simulink model "zynq_7000_tutorial_3"  (R2023b)
settings: Solver=FixedStepDiscrete  StartTime=0.0  StopTime=10.0  RelTol=1e-3
PostLoadFcn:
  | zynq7000.setModelProperties(bdroot)
undefined symbols (not defined in the file): AXI_VDMA, B, cam_init, G, init_cam, out1, out2, out3, OV5640, PS_GPIO, PS_IIC, R, read_cam_rgb, ScuGicInterruptController, VideoOutput
libraries: waijung2_utilities_lib x2, deeplib x1, zynq7000_device_config_lib x1
Description:
  | This model is created using Waijung 2
  | (Version: 23.5a)
settings Model: Creator=Aimagin  LastModifiedBy=Chris
settings SolverCC: PositivePriorityOrder=on  AutoInsertRateTranBlk=on
settings OptimizationCC: DefaultParameterBehavior=Inlined  EnhancedBackFolding=on  PassReuseOutputArgsAs=Individual arguments  ZeroExternalMemoryAtStartup=off  ZeroInternalMemoryAtStartup=off  OptimizeBlockOrder=speed  DifferentSizesBufferReuse=on  OptimizationCustomize=off  EfficientTunableParamExpr=on
settings DebuggingCC: ParameterTunabilityLossMsg=error
settings HardwareCC: ProdBitPerPointer=32  ProdBitPerSizeT=32  ProdBitPerPtrDiffT=32  ProdLargestAtomicInteger=Long  ProdLargestAtomicFloat=Double  ProdWordSize=32  ProdHWDeviceType=ARM Compatible->ARM Cortex
settings ModelReferenceCC: EnableRefExpFcnMdlSchedulingChecks=on
settings SFSimCC: MATLABDynamicMemAlloc=off
settings RTWCC: Description=Waijung 2 ZYNQ7000 target  SystemTargetFile=zynq7000.tlc  TemplateMakefile=zynq7000.tmf  RetainRTWFile=on  TargetLang=C++  DLTargetLibrary=arm-compute  DLArmComputeArch=armv7
settings CodeAppCC: ForceParamTrailComments=on  IgnoreCustomStorageClasses=off  OperatorAnnotations=on  SimulinkDataObjDesc=on  SFDataObjDesc=on  InsertBlockDesc=on
settings STFCustomTargetCC: TargetLangStandard=C++11 (ISO)  MultiwordLength=256  GenerateSampleERTMain=on  ModelReferenceCompliant=off  CombineOutputUpdateFcns=on  ERTCustomFileBanners=on  SupportContinuousTime=off  SupportNonInlinedSFcns=off  RemoveResetFunc=on  SupportVariableSizeSignals=on  MATLABClassNameForMDSCustomization=Simulink.SoftwareTarget.ERTCustomization  SystemTargetFile=zynq7000.tlc
settings ERTTargetCC: TargetLangStandard=C++11 (ISO)  GenerateSampleERTMain=on  ModelReferenceCompliant=off  ParMdlRefBuildCompliant=off  CompOptLevelCompliant=off  ConcurrentExecutionCompliant=off  SupportVariableSizeSignals=on  ModelStepFunctionPrototypeControlCompliant=off  CPPClassGenCompliant=off  UseToolchainInfoCompliant=off  InlinedParameterPlacement=NonHierarchical  ERTSrcFileBannerTemplate=zynq7000_code_template.cgt  ERTHdrFileBannerTemplate=zynq7000_code_template.cgt  ERTDataSrcFileTemplate=zynq7000_code_template.cgt  ERTDataHdrFileTemplate=zynq7000_code_template.cgt  ERTCustomFileTemplate=zynq7000_file_process.tlc

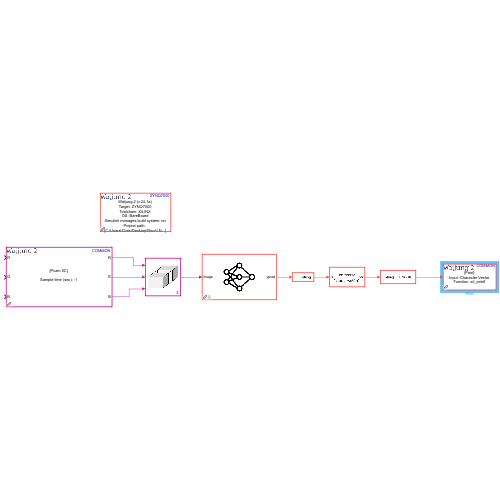
[thumbnail: Simulink's stored preview of the top-level diagram]
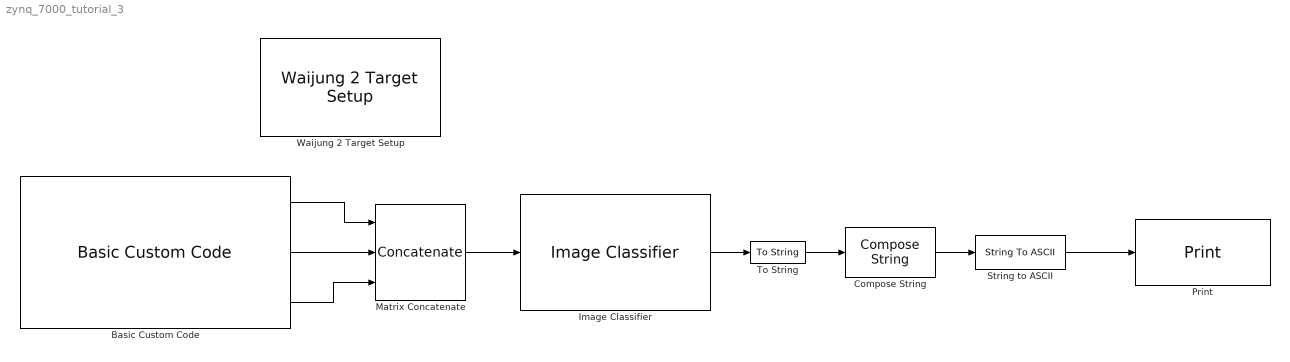
== system zynq_7000_tutorial_3 ==
  Basic Custom Code : waijung2_utilities_lib/Basic Custom Code  blockid=BasicCustomCode  maskdispname=Pcam 5C  inporttable={ 'R', 'uint8'; 'G', 'uint8'; 'B', 'uint8' }  outporttable={ 'R', 'uint8', '1280x720'; 'G', 'uint8', '1280x720'; 'B', 'uint8', '1280x720' }  inputporttype=uint8,uint8,uint8  cinputportlabel=R,G,B  cinputportlabelstr="[\"R\",\"G\",\"B\"]"  inputportcount=3  inputporttypeid="[3  3  3]"  outputporttype=uint8:1280x720,uint8:1280x720,uint8:1280x720  coutputportlabel=R,G,B  coutputportlabelstr="[\"R\",\"G\",\"B\"]"  outputportcount=3  outputporttypeid="[3  3  3]"  filepath="pwd,\"custom_lib\""  filenames=AXI_VDMA.c,AXI_VDMA.h,cam_init.c,cam_init.h,OV5640.c,OV5640.h,PS_GPIO.c,PS_GPIO.h,PS_IIC.c,PS_IIC.h,ScuGicInterruptController.h,VideoOutput.c,VideoOutput.h  incfilestrarray="[\"AXI_VDMA.h\",\"cam_init.h\",\"OV5640.h\",\"PS_GPIO.h\",\"PS_IIC.h\",\"ScuGicInterruptController.h\",\"VideoOutput.h\"]"  files=C:\Users\Chris\Desktop\RiscV-NPU-DualCore\NPU\custom_lib\AXI_VDMA.c,C:\Users\Chris\Desktop\RiscV-NPU-DualCore\NPU\custom_lib\AXI_VDMA.h,C:\Users\Chris\Desktop\RiscV-NPU-DualCore\NPU\custom_lib\cam_init.c,C:\Users\Chris\Desktop\RiscV-NPU-DualCore\NPU\custom_lib\cam_init.h,C:\Users\Chris\Desktop\RiscV-NPU-DualCore\NPU\custom_lib\OV5640.c,C:\Users\Chris\Desktop\RiscV-NPU-DualCore\NPU\custom_lib\OV5640.h,C:\Users\Chris\Desktop\RiscV-NPU-DualCore\NPU\custom_lib\PS_GPIO.c,C:\Users\Chris\Desktop\RiscV-NPU-DualCore\NPU\custom_lib\PS_GPIO.h,C:\Users\Chris\Desktop\RiscV-NPU-DualCore\NPU\custom_lib\PS_IIC.c,C:\Users\Chris\Desktop\RiscV-NPU-DualCore\NPU\custom_lib\PS_IIC.h,C:\Users\Chris\Desktop\RiscV-NPU-DualCore\NPU\custom_lib\ScuGicInterruptController.h,C:\Users\Chris\Desktop\RiscV-NPU-DualCore\NPU\custom_lib\VideoOutput.c,C:\Users\Chris\Desktop\RiscV-NPU-DualCore\NPU\custom_lib\VideoOutput.h  initialfuncallstr=init_cam();  outputfuncallstr=read_cam_rgb(out1, out2, out3);  inputportdiminfo="[1  1  1  3;1  1  1  3;1  1  1  3]"  outputportdiminfo="[1280     720  921600       3;1280     720  921600       3;1280     720  921600       3]"  enablecustomportlabel=on  sampletime=-1
      settings: SourceProductName=Waijung 2 Blockset
  Compose String : ComposeString  Format="\"label: %s\\r\\n\""
  Image Classifier : deeplib/Image Classifier  Network=Network from MATLAB function  NetworkFunction=mobilenetv2  NetworkFilePath=untitled.mat  MiniBatchSize=128  ResizeInput=on  Classification=on  Predictions=off  ForceInterpretedSim=off  PredictMode=All probabilities and labels  K=5
  Matrix Concatenate : Concatenate  NumInputs=3  Mode=Multidimensional array  ConcatenateDimension=3
  Print : waijung2_utilities_lib/Print  printfcn=xil_printf  strinput=Character Vector  sampletime=-1  blockid=Print  sampletimestr=2
      settings: SourceProductName=Waijung 2 Blockset
  String to ASCII : StringToASCII  OutputVectorSize=65
  To String : ToString
  Waijung 2 Target Setup : zynq7000_device_config_lib/Waijung 2 Target Setup  toolchain=XILINX  os=BareBoard  os_def=standalone  coreid=ps7_cortexa9_0  sampletime=-1  xilinxtoolpath=F:\  simulink_managebuildsystem=on  projectpath=C:\Users\Chris\Desktop\RiscV-NPU-DualCore\NPU  enableoverrun=off  gpiopin=7  digitalinoutcount=0  programto=SD card  flashtype=qspi_single  regenerate_platform=off  buildoptions=Deploy to hardware  buildoptionsdef=Deploy to hardware  blockid=Waijung2TargetSetup  target=ZYNQ7000  waijungversion=24.1a  defaultstacksize=2048  basepriority=0  highestpriority=8  generate_baserate_task=on  freertostickrate=100  freertosheap=65536  zynq7000flashsize=4MB  xsafilemode=Custom XSA file  xsapath=C:\Users\Chris\Downloads\zynq_7000_tutorial3.xsa  stdindef=none  stdoutdef=none  stacksize=0x3000000  heapsize=0x9900000  cpufreq=666666687  cominterface=Serial  serialdeviceid=XPAR_PS7_UART_0_DEVICE_ID  serialport=20  baudrate=115200  tcpdeviceid=XPAR_PS7_ETHERNET_0_DEVICE_ID  deviceip=192.168.1.10  targetnetmask=255.255.255.0  targetgateway=192.168.1.1  ipport=256  targetmac=00-0a-35-00-01-02  targetmacdef="[\"0x00\",\"0x0a\",\"0x35\",\"0x00\",\"0x01\",\"0x02\"]"  targetipdef=192,168,1,10  targetmaskdef=255,255,255,0  targetgatewaydef=192,168,1,1  exttimeout=10  extverbose=off
      settings: SourceProductName=Waijung 2 Blockset
  wires:
  Basic Custom Code/1 -> Matrix Concatenate/1
  Basic Custom Code/2 -> Matrix Concatenate/2
  Basic Custom Code/3 -> Matrix Concatenate/3
  Matrix Concatenate/1 -> Image Classifier/1
  Image Classifier/1 -> To String/1
  To String/1 -> Compose String/1
  Compose String/1 -> String to ASCII/1
  String to ASCII/1 -> Print/1
